simulink model "certus2"  (Simulink 7.1)
settings: Solver=VariableStepDiscrete  StartTime=0.0  StopTime=inf  MaxStep=0.2  RelTol=1e-3
libraries: SimvtkRenderingLibrary x9, SimvtkGraphicsLibrary x2, SimvtkOpenIGTLibrary x2, SimvtkCommonLibrary x1, SimvtkHybridLibrary x1
settings Model: Creator=acampi  LastModifiedBy=Administrator

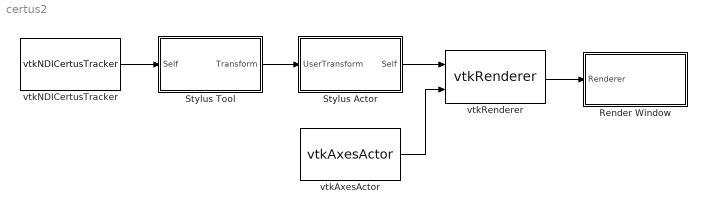
== system certus2 ==
  Render Window : Subsystem
  Stylus Actor : Subsystem
  Stylus Tool : Subsystem
  vtkAxesActor : SimvtkHybridLibrary/vtkAxesActor  VTKInputSelf=off  VTKInputUserDefinedShaft=off  VTKInputUserDefinedTip=off  VTKInputUserMatrix=off  VTKInputUserTransform=off  AxisLabelsInputIndicator=Use Default  VTKParamAxisLabels=0  ConeRadiusInputIndicator=Use Default  VTKParamConeRadius=0  ConeRadiusMaxValueInputIndicator=off  VTKParamConeRadiusMaxValue=0  ConeRadiusMinValueInputIndicator=off  VTKParamConeRadiusMinValue=0  ConeResolutionInputIndicator=Use Default  VTKParamConeResolution=0  ConeResolutionMaxValueInputIndicator=off  VTKParamConeResolutionMaxValue=0  ConeResolutionMinValueInputIndicator=off  VTKParamConeResolutionMinValue=0  CylinderRadiusInputIndicator=Use Default  VTKParamCylinderRadius=0  CylinderRadiusMaxValueInputIndicator=off  VTKParamCylinderRadiusMaxValue=0  CylinderRadiusMinValueInputIndicator=off  VTKParamCylinderRadiusMinValue=0  CylinderResolutionInputIndicator=Use Default  VTKParamCylinderResolution=0  CylinderResolutionMaxValueInputIndicator=off  VTKParamCylinderResolutionMaxValue=0  CylinderResolutionMinValueInputIndicator=off  VTKParamCylinderResolutionMinValue=0  DragableInputIndicator=Use Default  VTKParamDragable=0  IsIdentityInputIndicator=off  VTKParamIsIdentity=0  LengthInputIndicator=off  VTKParamLength=0  NormalizedLabelPositionInputIndicator=Use Default  VTKParamNormalizedLabelPosition=[0,0,0]  NormalizedShaftLengthInputIndicator=Use Default  VTKParamNormalizedShaftLength=[50,50,50]  NormalizedTipLengthInputIndicator=Use Default  VTKParamNormalizedTipLength=[0,0,0]  NumberOfPathsInputIndicator=off  VTKParamNumberOfPaths=0  OrientationInputIndicator=Use Default  VTKParamOrientation=[0,0,0]  OriginInputIndicator=Use Default  VTKParamOrigin=[0,0,0]  PickableInputIndicator=Use Default  VTKParamPickable=0  PositionInputIndicator=Use Default  VTKParamPosition=[0,0,0]  RedrawMTimeInputIndicator=off  VTKParamRedrawMTime=0  ScaleInputIndicator=Use Default  VTKParamScale=[0,0,0]  ShaftTypeInputIndicator=Use Default  VTKParamShaftType=0  SphereRadiusInputIndicator=Use Default  VTKParamSphereRadius=0  SphereRadiusMaxValueInputIndicator=off  VTKParamSphereRadiusMaxValue=0  SphereRadiusMinValueInputIndicator=off  VTKParamSphereRadiusMinValue=0  SphereResolutionInputIndicator=Use Default  VTKParamSphereResolution=0  SphereResolutionMaxValueInputIndicator=off  VTKParamSphereResolutionMaxValue=0  SphereResolutionMinValueInputIndicator=off  VTKParamSphereResolutionMinValue=0  TipTypeInputIndicator=Use Default  VTKParamTipType=0  TotalLengthInputIndicator=As Parameter  VTKParamTotalLength=[100,100,100]  UserTransformMatrixMTimeInputIndicator=off  VTKParamUserTransformMatrixMTime=0  VisibilityInputIndicator=Use Default  VTKParamVisibility=0  XAxisLabelTextInputIndicator=Use Default  VTKParamXAxisLabelText=0  YAxisLabelTextInputIndicator=Use Default  VTKParamYAxisLabelText=0  ZAxisLabelTextInputIndicator=Use Default  VTKParamZAxisLabelText=0  VTKOutputSelf=on  VTKOutputMatrix=off  VTKOutputNextPath=off  VTKOutputXAxisCaptionActor2D=off  VTKOutputXAxisShaftProperty=off  VTKOutputXAxisTipProperty=off  VTKOutputYAxisCaptionActor2D=off  VTKOutputYAxisShaftProperty=off  VTKOutputYAxisTipProperty=off  VTKOutputZAxisCaptionActor2D=off  VTKOutputZAxisShaftProperty=off  VTKOutputZAxisTipProperty=off
  vtkNDICertusTracker : SimvtkOpenIGTLibrary/vtkNDICertusTracker  VTKInputSelf=off  VTKInputTool=off  VTKInputWorldCalibrationMatrix=off  InternalUpdateRateInputIndicator=off  VTKParamInternalUpdateRate=0  NetworkPortInputIndicator=Use Default  VTKParamNetworkPort=0  NumberOfToolsInputIndicator=off  VTKParamNumberOfTools=0  ReferenceToolInputIndicator=As Parameter  VTKParamReferenceTool=1  RemoteAddressInputIndicator=Use Default  VTKParamRemoteAddress=0  ServerModeInputIndicator=Use Default  VTKParamServerMode=0  ToolLEDInputIndicator=Use Default  VTKParamToolLED=[0,0,0]  TrackingInputIndicator=As Parameter  VTKParamTracking=1  UpdateTimeStampInputIndicator=off  VTKParamUpdateTimeStamp=0  VTKOutputSelf=off  VTKOutputSocketCommunicator=off  VTKOutputTool0=on  VTKOutputTool1=off  VTKOutputTool2=off
  vtkRenderer : SimvtkRenderingLibrary/vtkRenderer  VTKInputSelf=off  VTKInputActiveCamera=off  VTKInputActor=2  VTKInputActor2D=0  VTKInputCuller=0  VTKInputLight=0  VTKInputProp=0  VTKInputViewProp=0  VTKInputVolume=0  AllocatedRenderTimeInputIndicator=Use Default  VTKParamAllocatedRenderTime=0  AmbientInputIndicator=Use Default  VTKParamAmbient=[0,0,0]  AspectInputIndicator=Use Default  VTKParamAspect=[0,0]  AutomaticLightCreationInputIndicator=Use Default  VTKParamAutomaticLightCreation=0  BackgroundInputIndicator=Use Default  VTKParamBackground=[0,0,0]  Background2InputIndicator=Use Default  VTKParamBackground2=[0,0,0]  BackingStoreInputIndicator=Use Default  VTKParamBackingStore=0  DisplayPointInputIndicator=Use Default  VTKParamDisplayPoint=[0,0,0]  DrawInputIndicator=Use Default  VTKParamDraw=0  EraseInputIndicator=Use Default  VTKParamErase=0  GradientBackgroundInputIndicator=Use Default  VTKParamGradientBackground=0  InteractiveInputIndicator=Use Default  VTKParamInteractive=0  IsPickingInputIndicator=off  VTKParamIsPicking=0  LastRenderTimeInSecondsInputIndicator=off  VTKParamLastRenderTimeInSeconds=0  LastRenderingUsedDepthPeelingInputIndicator=off  VTKParamLastRenderingUsedDepthPeeling=0  LayerInputIndicator=Use Default  VTKParamLayer=0  LightFollowCameraInputIndicator=Use Default  VTKParamLightFollowCamera=0  MaximumNumberOfPeelsInputIndicator=Use Default  VTKParamMaximumNumberOfPeels=0  NearClippingPlaneToleranceInputIndicator=Use Default  VTKParamNearClippingPlaneTolerance=0  NearClippingPlaneToleranceMaxValueInputIndicator=off  VTKParamNearClippingPlaneToleranceMaxValue=0  NearClippingPlaneToleranceMinValueInputIndicator=off  VTKParamNearClippingPlaneToleranceMinValue=0  NumberOfPropsRenderedInputIndicator=off  VTKParamNumberOfPropsRendered=0  OcclusionRatioInputIndicator=Use Default  VTKParamOcclusionRatio=0  OcclusionRatioMaxValueInputIndicator=off  VTKParamOcclusionRatioMaxValue=0  OcclusionRatioMinValueInputIndicator=off  VTKParamOcclusionRatioMinValue=0  PickHeightInputIndicator=off  VTKParamPickHeight=0  PickWidthInputIndicator=off  VTKParamPickWidth=0  PickXInputIndicator=off  VTKParamPickX=0  PickX1InputIndicator=off  VTKParamPickX1=0  PickX2InputIndicator=off  VTKParamPickX2=0  PickYInputIndicator=off  VTKParamPickY=0  PickY1InputIndicator=off  VTKParamPickY1=0  PickY2InputIndicator=off  VTKParamPickY2=0  PickedZInputIndicator=off  VTKParamPickedZ=0  PixelAspectInputIndicator=Use Default  VTKParamPixelAspect=[0,0]  TiledAspectRatioInputIndicator=off  VTKParamTiledAspectRatio=0  TimeFactorInputIndicator=off  VTKParamTimeFactor=0  TwoSidedLightingInputIndicator=Use Default  VTKParamTwoSidedLighting=0  UseDepthPeelingInputIndicator=Use Default  VTKParamUseDepthPeeling=0  ViewPointInputIndicator=Use Default  VTKParamViewPoint=[0,0,0]  ViewportInputIndicator=Use Default  VTKParamViewport=[0,0,0,0]  WorldPointInputIndicator=Use Default  VTKParamWorldPoint=[0,0,0,0]  VTKOutputSelf=on  VTKOutputActors=off  VTKOutputActors2D=off  VTKOutputCullers=off  VTKOutputLights=off  VTKOutputPickResultProps=off  VTKOutputProps=off  VTKOutputVTKWindow=off  VTKOutputViewProps=off  VTKOutputVolumes=off
  wires:
  Stylus Tool/1(Transform) -> Stylus Actor/1(UserTransform)
  vtkNDICertusTracker/1 -> Stylus Tool/1(Self)
  vtkRenderer/1 -> Render Window/1(Renderer)
  Stylus Actor/1(Self) -> vtkRenderer/1
  vtkAxesActor/1 -> vtkRenderer/2

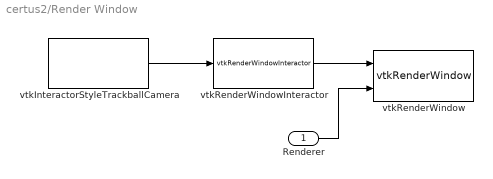
== system certus2/Render Window ==
  Renderer : Inport  OutDataType=sfix(16)  OutScaling=2^0
  vtkInteractorStyleTrackballCamera : SimvtkRenderingLibrary/vtkInteractorStyleTrackballCamera  VTKInputSelf=off  VTKInputCurrentRenderer=off  VTKInputDefaultRenderer=off  VTKInputInteractor=off  AutoAdjustCameraClippingRangeInputIndicator=Use Default  VTKParamAutoAdjustCameraClippingRange=0  AutoAdjustCameraClippingRangeMaxValueInputIndicator=off  VTKParamAutoAdjustCameraClippingRangeMaxValue=0  AutoAdjustCameraClippingRangeMinValueInputIndicator=off  VTKParamAutoAdjustCameraClippingRangeMinValue=0  EnabledInputIndicator=Use Default  VTKParamEnabled=0  HandleObserversInputIndicator=Use Default  VTKParamHandleObservers=0  KeyPressActivationInputIndicator=Use Default  VTKParamKeyPressActivation=0  KeyPressActivationValueInputIndicator=Use Default  VTKParamKeyPressActivationValue=0  MotionFactorInputIndicator=Use Default  VTKParamMotionFactor=0  MouseWheelMotionFactorInputIndicator=Use Default  VTKParamMouseWheelMotionFactor=0  PickColorInputIndicator=Use Default  VTKParamPickColor=[0,0,0]  PriorityInputIndicator=Use Default  VTKParamPriority=0  PriorityMaxValueInputIndicator=off  VTKParamPriorityMaxValue=0  PriorityMinValueInputIndicator=off  VTKParamPriorityMinValue=0  StateInputIndicator=off  VTKParamState=0  TimerDurationInputIndicator=Use Default  VTKParamTimerDuration=0  TimerDurationMaxValueInputIndicator=off  VTKParamTimerDurationMaxValue=0  TimerDurationMinValueInputIndicator=off  VTKParamTimerDurationMinValue=0  UseTimersInputIndicator=Use Default  VTKParamUseTimers=0  VTKOutputSelf=on
  vtkRenderWindow : SimvtkRenderingLibrary/vtkRenderWindow  VTKInputSelf=off  VTKInputInteractor=on  VTKInputRenderer=1  AAFramesInputIndicator=Use Default  VTKParamAAFrames=0  AbortRenderInputIndicator=Use Default  VTKParamAbortRender=0  AlphaBitPlanesInputIndicator=Use Default  VTKParamAlphaBitPlanes=0  AnaglyphColorMaskInputIndicator=Use Default  VTKParamAnaglyphColorMask=[0,0]  AnaglyphColorSaturationInputIndicator=Use Default  VTKParamAnaglyphColorSaturation=0  AnaglyphColorSaturationMaxValueInputIndicator=off  VTKParamAnaglyphColorSaturationMaxValue=0  AnaglyphColorSaturationMinValueInputIndicator=off  VTKParamAnaglyphColorSaturationMinValue=0  BordersInputIndicator=Use Default  VTKParamBorders=0  CurrentCursorInputIndicator=Use Default  VTKParamCurrentCursor=0  CursorPositionInputIndicator=Use Default  VTKParamCursorPosition=[0,0]  DPIInputIndicator=Use Default  VTKParamDPI=0  DPIMaxValueInputIndicator=off  VTKParamDPIMaxValue=0  DPIMinValueInputIndicator=off  VTKParamDPIMinValue=0  DepthBufferSizeInputIndicator=off  VTKParamDepthBufferSize=0  DesiredUpdateRateInputIndicator=Use Default  VTKParamDesiredUpdateRate=0  DoubleBufferInputIndicator=Use Default  VTKParamDoubleBuffer=0  EraseInputIndicator=Use Default  VTKParamErase=0  EventPendingInputIndicator=off  VTKParamEventPending=0  FDFramesInputIndicator=Use Default  VTKParamFDFrames=0  FullScreenInputIndicator=Use Default  VTKParamFullScreen=0  InAbortCheckInputIndicator=Use Default  VTKParamInAbortCheck=0  IsPickingInputIndicator=Use Default  VTKParamIsPicking=0  LastGraphicErrorStringInputIndicator=off  VTKParamLastGraphicErrorString=0  LineSmoothingInputIndicator=Use Default  VTKParamLineSmoothing=0  MappedInputIndicator=Use Default  VTKParamMapped=0  MultiSamplesInputIndicator=Use Default  VTKParamMultiSamples=0  NeverRenderedInputIndicator=off  VTKParamNeverRendered=0  NextWindowInfoInputIndicator=Use Default  VTKParamNextWindowInfo=0  NumberOfLayersInputIndicator=Use Default  VTKParamNumberOfLayers=0  NumberOfLayersMaxValueInputIndicator=off  VTKParamNumberOfLayersMaxValue=0  NumberOfLayersMinValueInputIndicator=off  VTKParamNumberOfLayersMinValue=0  OffScreenRenderingInputIndicator=Use Default  VTKParamOffScreenRendering=0  ParentInfoInputIndicator=Use Default  VTKParamParentInfo=0  PointSmoothingInputIndicator=Use Default  VTKParamPointSmoothing=0  PolygonSmoothingInputIndicator=Use Default  VTKParamPolygonSmoothing=0  PositionInputIndicator=Use Default  VTKParamPosition=[0,0]  RenderLibraryInputIndicator=off  VTKParamRenderLibrary=0  ReportGraphicErrorsInputIndicator=Use Default  VTKParamReportGraphicErrors=0  SizeInputIndicator=Use Default  VTKParamSize=[0,0]  StencilCapableInputIndicator=Use Default  VTKParamStencilCapable=0  StereoCapableWindowInputIndicator=Use Default  VTKParamStereoCapableWindow=0  StereoRenderInputIndicator=Use Default  VTKParamStereoRender=0  StereoTypeInputIndicator=Use Default  VTKParamStereoType=0  StereoTypeAsStringInputIndicator=off  VTKParamStereoTypeAsString=0  SubFramesInputIndicator=Use Default  VTKParamSubFrames=0  SwapBuffersInputIndicator=Use Default  VTKParamSwapBuffers=0  TileScaleInputIndicator=Use Default  VTKParamTileScale=[0,0]  TileViewportInputIndicator=Use Default  VTKParamTileViewport=[0,0,0,0]  WindowInfoInputIndicator=Use Default  VTKParamWindowInfo=0  WindowNameInputIndicator=Use Default  VTKParamWindowName=0  VTKOutputSelf=off  VTKOutputPainterDeviceAdapter=off  VTKOutputRenderers=off
  vtkRenderWindowInteractor : SimvtkRenderingLibrary/vtkRenderWindowInteractor  VTKInputSelf=off  VTKInputInteractorStyle=on  VTKInputPicker=off  VTKInputRenderWindow=off  AltKeyInputIndicator=Use Default  VTKParamAltKey=0  ControlKeyInputIndicator=Use Default  VTKParamControlKey=0  DesiredUpdateRateInputIndicator=Use Default  VTKParamDesiredUpdateRate=0  DesiredUpdateRateMaxValueInputIndicator=off  VTKParamDesiredUpdateRateMaxValue=0  DesiredUpdateRateMinValueInputIndicator=off  VTKParamDesiredUpdateRateMinValue=0  DollyInputIndicator=Use Default  VTKParamDolly=0  EnabledInputIndicator=off  VTKParamEnabled=0  EventPositionInputIndicator=Use Default  VTKParamEventPosition=[0,0]  EventPositionFlipYInputIndicator=Use Default  VTKParamEventPositionFlipY=[0,0]  EventSizeInputIndicator=Use Default  VTKParamEventSize=[0,0]  InitializedInputIndicator=off  VTKParamInitialized=0  KeyCodeInputIndicator=Use Default  VTKParamKeyCode=0  KeySymInputIndicator=Use Default  VTKParamKeySym=0  LastEventPositionInputIndicator=Use Default  VTKParamLastEventPosition=[0,0]  LightFollowCameraInputIndicator=Use Default  VTKParamLightFollowCamera=0  NumberOfFlyFramesInputIndicator=Use Default  VTKParamNumberOfFlyFrames=0  NumberOfFlyFramesMaxValueInputIndicator=off  VTKParamNumberOfFlyFramesMaxValue=0  NumberOfFlyFramesMinValueInputIndicator=off  VTKParamNumberOfFlyFramesMinValue=0  RepeatCountInputIndicator=Use Default  VTKParamRepeatCount=0  ShiftKeyInputIndicator=Use Default  VTKParamShiftKey=0  SizeInputIndicator=Use Default  VTKParamSize=[0,0]  StillUpdateRateInputIndicator=Use Default  VTKParamStillUpdateRate=0  StillUpdateRateMaxValueInputIndicator=off  VTKParamStillUpdateRateMaxValue=0  StillUpdateRateMinValueInputIndicator=off  VTKParamStillUpdateRateMinValue=0  TimerDurationInputIndicator=Use Default  VTKParamTimerDuration=0  TimerDurationMaxValueInputIndicator=off  VTKParamTimerDurationMaxValue=0  TimerDurationMinValueInputIndicator=off  VTKParamTimerDurationMinValue=0  TimerEventDurationInputIndicator=Use Default  VTKParamTimerEventDuration=0  TimerEventIdInputIndicator=Use Default  VTKParamTimerEventId=0  TimerEventPlatformIdInputIndicator=Use Default  VTKParamTimerEventPlatformId=0  TimerEventTypeInputIndicator=Use Default  VTKParamTimerEventType=0  VTKOutputSelf=on  VTKOutputObserverMediator=off
  wires:
  vtkRenderWindowInteractor/1 -> vtkRenderWindow/1
  vtkInteractorStyleTrackballCamera/1 -> vtkRenderWindowInteractor/1
  Renderer/1 -> vtkRenderWindow/2

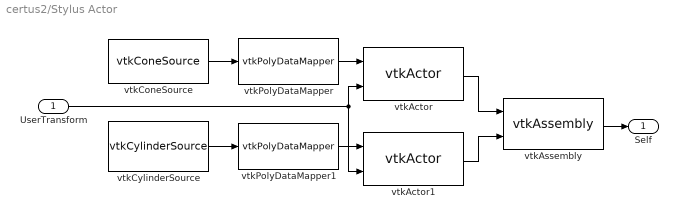
== system certus2/Stylus Actor ==
  UserTransform : Inport  OutDataType=sfix(16)  OutScaling=2^0
  vtkActor : SimvtkRenderingLibrary/vtkActor  VTKInputSelf=off  VTKInputBackfaceProperty=off  VTKInputMapper=on  VTKInputProperty=off  VTKInputTexture=off  VTKInputUserMatrix=off  VTKInputUserTransform=on  DragableInputIndicator=Use Default  VTKParamDragable=0  IsIdentityInputIndicator=off  VTKParamIsIdentity=0  LengthInputIndicator=off  VTKParamLength=0  NumberOfPartsInputIndicator=off  VTKParamNumberOfParts=0  NumberOfPathsInputIndicator=off  VTKParamNumberOfPaths=0  OrientationInputIndicator=Use Default  VTKParamOrientation=[0,0,0]  OriginInputIndicator=Use Default  VTKParamOrigin=[0,0,0]  PickableInputIndicator=Use Default  VTKParamPickable=0  PositionInputIndicator=Use Default  VTKParamPosition=[0,0,0]  RedrawMTimeInputIndicator=off  VTKParamRedrawMTime=0  ScaleInputIndicator=Use Default  VTKParamScale=[0,0,0]  UserTransformMatrixMTimeInputIndicator=off  VTKParamUserTransformMatrixMTime=0  VisibilityInputIndicator=Use Default  VTKParamVisibility=0  VTKOutputSelf=on  VTKOutputMatrix=off  VTKOutputNextPart=off  VTKOutputNextPath=off
  vtkActor1 : SimvtkRenderingLibrary/vtkActor  VTKInputSelf=off  VTKInputBackfaceProperty=off  VTKInputMapper=on  VTKInputProperty=off  VTKInputTexture=off  VTKInputUserMatrix=off  VTKInputUserTransform=on  DragableInputIndicator=Use Default  VTKParamDragable=0  IsIdentityInputIndicator=off  VTKParamIsIdentity=0  LengthInputIndicator=off  VTKParamLength=0  NumberOfPartsInputIndicator=off  VTKParamNumberOfParts=0  NumberOfPathsInputIndicator=off  VTKParamNumberOfPaths=0  OrientationInputIndicator=As Parameter  VTKParamOrientation=[0,0,90]  OriginInputIndicator=As Parameter  VTKParamOrigin=[0,0,0]  PickableInputIndicator=Use Default  VTKParamPickable=0  PositionInputIndicator=Use Default  VTKParamPosition=[0,0,0]  RedrawMTimeInputIndicator=off  VTKParamRedrawMTime=0  ScaleInputIndicator=Use Default  VTKParamScale=[0,0,0]  UserTransformMatrixMTimeInputIndicator=off  VTKParamUserTransformMatrixMTime=0  VisibilityInputIndicator=Use Default  VTKParamVisibility=0  VTKOutputSelf=on  VTKOutputMatrix=off  VTKOutputNextPart=off  VTKOutputNextPath=off
  vtkAssembly : SimvtkRenderingLibrary/vtkAssembly  VTKInputSelf=off  VTKInputPart=2  VTKInputUserMatrix=off  VTKInputUserTransform=off  DragableInputIndicator=Use Default  VTKParamDragable=0  IsIdentityInputIndicator=off  VTKParamIsIdentity=0  LengthInputIndicator=off  VTKParamLength=0  NumberOfPathsInputIndicator=off  VTKParamNumberOfPaths=0  OrientationInputIndicator=Use Default  VTKParamOrientation=[0,0,0]  OriginInputIndicator=Use Default  VTKParamOrigin=[0,0,0]  PickableInputIndicator=Use Default  VTKParamPickable=0  PositionInputIndicator=Use Default  VTKParamPosition=[0,0,0]  RedrawMTimeInputIndicator=off  VTKParamRedrawMTime=0  ScaleInputIndicator=Use Default  VTKParamScale=[0,0,0]  UserTransformMatrixMTimeInputIndicator=off  VTKParamUserTransformMatrixMTime=0  VisibilityInputIndicator=Use Default  VTKParamVisibility=0  VTKOutputSelf=on  VTKOutputMatrix=off  VTKOutputNextPath=off  VTKOutputParts=off
  vtkConeSource : SimvtkGraphicsLibrary/vtkConeSource  VTKInputSelf=off  AngleInputIndicator=Use Default  VTKParamAngle=0  CappingInputIndicator=Use Default  VTKParamCapping=0  CenterInputIndicator=As Parameter  VTKParamCenter=[-5,0,0]  DirectionInputIndicator=As Parameter  VTKParamDirection=[1,0,0]  HeightInputIndicator=As Parameter  VTKParamHeight=10  HeightMaxValueInputIndicator=off  VTKParamHeightMaxValue=0  HeightMinValueInputIndicator=off  VTKParamHeightMinValue=0  RadiusInputIndicator=As Parameter  VTKParamRadius=2  RadiusMaxValueInputIndicator=off  VTKParamRadiusMaxValue=0  RadiusMinValueInputIndicator=off  VTKParamRadiusMinValue=0  ResolutionInputIndicator=Use Default  VTKParamResolution=0  ResolutionMaxValueInputIndicator=off  VTKParamResolutionMaxValue=0  ResolutionMinValueInputIndicator=off  VTKParamResolutionMinValue=0  VTKOutputSelf=off
  vtkCylinderSource : SimvtkGraphicsLibrary/vtkCylinderSource  VTKInputSelf=off  CappingInputIndicator=As Parameter  VTKParamCapping=1  CenterInputIndicator=As Parameter  VTKParamCenter=[0,60,0]  HeightInputIndicator=As Parameter  VTKParamHeight=100  HeightMaxValueInputIndicator=off  VTKParamHeightMaxValue=0  HeightMinValueInputIndicator=off  VTKParamHeightMinValue=0  RadiusInputIndicator=As Parameter  VTKParamRadius=2  RadiusMaxValueInputIndicator=off  VTKParamRadiusMaxValue=0  RadiusMinValueInputIndicator=off  VTKParamRadiusMinValue=0  ResolutionInputIndicator=Use Default  VTKParamResolution=0  ResolutionMaxValueInputIndicator=off  VTKParamResolutionMaxValue=0  ResolutionMinValueInputIndicator=off  VTKParamResolutionMinValue=0  VTKOutputSelf=off
  vtkPolyDataMapper : SimvtkRenderingLibrary/vtkPolyDataMapper  VTKInputSelf=off  VTKInputClippingPlane=0  VTKInputClippingPlanes=off  VTKInputLookupTable=off  ArrayAccessModeInputIndicator=off  VTKParamArrayAccessMode=0  ArrayComponentInputIndicator=off  VTKParamArrayComponent=0  ArrayIdInputIndicator=off  VTKParamArrayId=0  ArrayNameInputIndicator=off  VTKParamArrayName=0  ColorModeInputIndicator=Use Default  VTKParamColorMode=0  ColorModeAsStringInputIndicator=off  VTKParamColorModeAsString=0  GhostLevelInputIndicator=Use Default  VTKParamGhostLevel=0  ImmediateModeRenderingInputIndicator=Use Default  VTKParamImmediateModeRendering=0  InterpolateScalarsBeforeMappingInputIndicator=Use Default  VTKParamInterpolateScalarsBeforeMapping=0  LengthInputIndicator=off  VTKParamLength=0  NumberOfPiecesInputIndicator=Use Default  VTKParamNumberOfPieces=0  NumberOfSubPiecesInputIndicator=Use Default  VTKParamNumberOfSubPieces=0  PieceInputIndicator=Use Default  VTKParamPiece=0  RenderTimeInputIndicator=Use Default  VTKParamRenderTime=0  ScalarMaterialModeInputIndicator=Use Default  VTKParamScalarMaterialMode=0  ScalarMaterialModeAsStringInputIndicator=off  VTKParamScalarMaterialModeAsString=0  ScalarModeInputIndicator=Use Default  VTKParamScalarMode=0  ScalarModeAsStringInputIndicator=off  VTKParamScalarModeAsString=0  ScalarRangeInputIndicator=Use Default  VTKParamScalarRange=[0,0]  ScalarVisibilityInputIndicator=Use Default  VTKParamScalarVisibility=0  StaticInputIndicator=Use Default  VTKParamStatic=0  TimeToDrawInputIndicator=off  VTKParamTimeToDraw=0  UseLookupTableScalarRangeInputIndicator=Use Default  VTKParamUseLookupTableScalarRange=0  VTKOutputSelf=on
  vtkPolyDataMapper1 : SimvtkRenderingLibrary/vtkPolyDataMapper  VTKInputSelf=off  VTKInputClippingPlane=0  VTKInputClippingPlanes=off  VTKInputLookupTable=off  ArrayAccessModeInputIndicator=off  VTKParamArrayAccessMode=0  ArrayComponentInputIndicator=off  VTKParamArrayComponent=0  ArrayIdInputIndicator=off  VTKParamArrayId=0  ArrayNameInputIndicator=off  VTKParamArrayName=0  ColorModeInputIndicator=Use Default  VTKParamColorMode=0  ColorModeAsStringInputIndicator=off  VTKParamColorModeAsString=0  GhostLevelInputIndicator=Use Default  VTKParamGhostLevel=0  ImmediateModeRenderingInputIndicator=Use Default  VTKParamImmediateModeRendering=0  InterpolateScalarsBeforeMappingInputIndicator=Use Default  VTKParamInterpolateScalarsBeforeMapping=0  LengthInputIndicator=off  VTKParamLength=0  NumberOfPiecesInputIndicator=Use Default  VTKParamNumberOfPieces=0  NumberOfSubPiecesInputIndicator=Use Default  VTKParamNumberOfSubPieces=0  PieceInputIndicator=Use Default  VTKParamPiece=0  RenderTimeInputIndicator=Use Default  VTKParamRenderTime=0  ScalarMaterialModeInputIndicator=Use Default  VTKParamScalarMaterialMode=0  ScalarMaterialModeAsStringInputIndicator=off  VTKParamScalarMaterialModeAsString=0  ScalarModeInputIndicator=Use Default  VTKParamScalarMode=0  ScalarModeAsStringInputIndicator=off  VTKParamScalarModeAsString=0  ScalarRangeInputIndicator=Use Default  VTKParamScalarRange=[0,0]  ScalarVisibilityInputIndicator=Use Default  VTKParamScalarVisibility=0  StaticInputIndicator=Use Default  VTKParamStatic=0  TimeToDrawInputIndicator=off  VTKParamTimeToDraw=0  UseLookupTableScalarRangeInputIndicator=Use Default  VTKParamUseLookupTableScalarRange=0  VTKOutputSelf=on
  Self : Outport  OutDataType=sfix(16)  OutScaling=2^0
  wires:
  vtkConeSource/1 -> vtkPolyDataMapper/1
  vtkPolyDataMapper/1 -> vtkActor/1
  UserTransform/1 -> vtkActor/2, vtkActor1/2
  vtkAssembly/1 -> Self/1
  vtkCylinderSource/1 -> vtkPolyDataMapper1/1
  vtkPolyDataMapper1/1 -> vtkActor1/1
  vtkActor/1 -> vtkAssembly/1
  vtkActor1/1 -> vtkAssembly/2

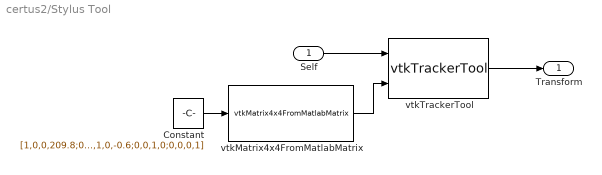
== system certus2/Stylus Tool ==
  Self : Inport  OutDataType=sfix(16)  OutScaling=2^0
  Constant : Constant  Value=[1,0,0,209.8;0,1,0,-0.6;0,0,1,0;0,0,0,1]  VectorParams1D=off  OutDataType=sfix(16)  OutScaling=2^0
  vtkMatrix4x4FromMatlabMatrix : SimvtkCommonLibrary/vtkMatrix4x4FromMatlabMatrix
  vtkTrackerTool : SimvtkOpenIGTLibrary/vtkTrackerTool  VTKInputSelf=on  VTKInputCalibrationMatrix=on  FlagsInputIndicator=off  VTKParamFlags=0  LED1InputIndicator=Use Default  VTKParamLED1=0  LED2InputIndicator=Use Default  VTKParamLED2=0  LED3InputIndicator=Use Default  VTKParamLED3=0  TimeStampInputIndicator=off  VTKParamTimeStamp=0  ToolManufacturerInputIndicator=off  VTKParamToolManufacturer=0  ToolPartNumberInputIndicator=off  VTKParamToolPartNumber=0  ToolPortInputIndicator=off  VTKParamToolPort=0  ToolRevisionInputIndicator=off  VTKParamToolRevision=0  ToolSerialNumberInputIndicator=off  VTKParamToolSerialNumber=0  ToolTypeInputIndicator=off  VTKParamToolType=0  VTKOutputSelf=off  VTKOutputBuffer=off  VTKOutputTracker=off  VTKOutputTransform=on
  Transform : Outport  OutDataType=sfix(16)  OutScaling=2^0
  wires:
  Constant/1 -> vtkMatrix4x4FromMatlabMatrix/1
  vtkMatrix4x4FromMatlabMatrix/1 -> vtkTrackerTool/2
  Self/1 -> vtkTrackerTool/1
  vtkTrackerTool/1 -> Transform/1
